simulink model "New_Control_Law_I_3Axis"  (R2016a)
settings: configuration reference "AR_Drone_ConfigSet" (kept outside this file)
values from neighbouring files (symbols this model uses):
  Accel_Calib_Gain = Simulink.Parameter    [AR_DRONE_SCRIPT.m]
  Accel_Calib_Offset = Simulink.Parameter    [AR_DRONE_SCRIPT.m]
undefined symbols (not defined in the file or in its folder): Drone_StateModeType, Mag_Calib_Gain_Vector, Mag_Calib_Offset_Vector, Navigation, Navigation_KF_Lib, sigbuilder_block
libraries: simulink x16, vrlib x7, aerolibtransform2 x5, AR_Drone_Sensors x2, AR_Drone_Actuators x2, aerolibutil x2, dspnetwork x2
(part 3 of 3)

== system New_Control_Law_I_3Axis/Sensor  Telemetry/CheckSum_Correct_Pressure/CheckSum Correction/Generate Sample Holding Pulse/Transition Logic Detection ==
  Input : Inport
  Constant : Constant  Value=0
  Constant1 : Constant
  Logical Operator : Logic  AllPortsSameDT=off  OutDataTypeStr=boolean
  Relational Operator : RelationalOperator  Operator===  OutDataTypeStr=boolean
  Relational Operator1 : RelationalOperator  Operator===  OutDataTypeStr=boolean
  Unit Delay : UnitDelay  SampleTime=-1
  Transition Detect : Outport
  wires:
  Relational Operator1/1 -> Logical Operator/1
  Unit Delay/1 -> Relational Operator/1
  Input/1 -> Relational Operator1/2, Unit Delay/1
  Relational Operator/1 -> Logical Operator/2
  Constant/1 -> Relational Operator/2
  Constant1/1 -> Relational Operator1/1
  Logical Operator/1 -> Transition Detect/1  "Transition_Detect"

== system New_Control_Law_I_3Axis/Sensor  Telemetry/CheckSum_Correct_Temp/CheckSum Correction/Generate Sample Holding Pulse/Transition Logic Detection ==
  Input : Inport
  Constant : Constant  Value=0
  Constant1 : Constant
  Logical Operator : Logic  AllPortsSameDT=off  OutDataTypeStr=boolean
  Relational Operator : RelationalOperator  Operator===  OutDataTypeStr=boolean
  Relational Operator1 : RelationalOperator  Operator===  OutDataTypeStr=boolean
  Unit Delay : UnitDelay  SampleTime=-1
  Transition Detect : Outport
  wires:
  Relational Operator1/1 -> Logical Operator/1
  Unit Delay/1 -> Relational Operator/1
  Input/1 -> Relational Operator1/2, Unit Delay/1
  Relational Operator/1 -> Logical Operator/2
  Constant/1 -> Relational Operator/2
  Constant1/1 -> Relational Operator1/1
  Logical Operator/1 -> Transition Detect/1  "Transition_Detect"

== system New_Control_Law_I_3Axis/Navigation/CheckSum Pre-Processing/Accelerometer Processing/CheckSum Correction/Generate Sample Holding Pulse/Transition Logic Detection ==
  Input : Inport
  Constant : Constant  Value=0
  Constant1 : Constant
  Logical Operator : Logic  AllPortsSameDT=off  OutDataTypeStr=boolean
  Relational Operator : RelationalOperator  Operator===  OutDataTypeStr=boolean
  Relational Operator1 : RelationalOperator  Operator===  OutDataTypeStr=boolean
  Unit Delay : UnitDelay  SampleTime=-1
  Transition Detect : Outport
  wires:
  Logical Operator/1 -> Transition Detect/1  "Transition_Detect"
  Constant1/1 -> Relational Operator1/1
  Constant/1 -> Relational Operator/2
  Relational Operator/1 -> Logical Operator/2
  Input/1 -> Unit Delay/1, Relational Operator1/2
  Unit Delay/1 -> Relational Operator/1
  Relational Operator1/1 -> Logical Operator/1

== system New_Control_Law_I_3Axis/Navigation/CheckSum Pre-Processing/Magnetometer/CheckSum Correction/Generate Sample Holding Pulse/Transition Logic Detection ==
  Input : Inport
  Constant : Constant  Value=0
  Constant1 : Constant
  Logical Operator : Logic  AllPortsSameDT=off  OutDataTypeStr=boolean
  Relational Operator : RelationalOperator  Operator===  OutDataTypeStr=boolean
  Relational Operator1 : RelationalOperator  Operator===  OutDataTypeStr=boolean
  Unit Delay : UnitDelay  SampleTime=-1
  Transition Detect : Outport
  wires:
  Logical Operator/1 -> Transition Detect/1  "Transition_Detect"
  Constant1/1 -> Relational Operator1/1
  Constant/1 -> Relational Operator/2
  Relational Operator/1 -> Logical Operator/2
  Input/1 -> Unit Delay/1, Relational Operator1/2
  Unit Delay/1 -> Relational Operator/1
  Relational Operator1/1 -> Logical Operator/1

== system New_Control_Law_I_3Axis/Navigation/CheckSum Pre-Processing/RateGyro Processing/CheckSum Correction/Generate Sample Holding Pulse/Transition Logic Detection ==
  Input : Inport
  Constant : Constant  Value=0
  Constant1 : Constant
  Logical Operator : Logic  AllPortsSameDT=off  OutDataTypeStr=boolean
  Relational Operator : RelationalOperator  Operator===  OutDataTypeStr=boolean
  Relational Operator1 : RelationalOperator  Operator===  OutDataTypeStr=boolean
  Unit Delay : UnitDelay  SampleTime=-1
  Transition Detect : Outport
  wires:
  Logical Operator/1 -> Transition Detect/1  "Transition_Detect"
  Constant1/1 -> Relational Operator1/1
  Constant/1 -> Relational Operator/2
  Relational Operator/1 -> Logical Operator/2
  Input/1 -> Unit Delay/1, Relational Operator1/2
  Unit Delay/1 -> Relational Operator/1
  Relational Operator1/1 -> Logical Operator/1

== system New_Control_Law_I_3Axis/Navigation/CheckSum Pre-Processing/TempFilter/CheckSum Correction/Generate Sample Holding Pulse/Transition Logic Detection ==
  Input : Inport
  Constant : Constant  Value=0
  Constant1 : Constant
  Logical Operator : Logic  AllPortsSameDT=off  OutDataTypeStr=boolean
  Relational Operator : RelationalOperator  Operator===  OutDataTypeStr=boolean
  Relational Operator1 : RelationalOperator  Operator===  OutDataTypeStr=boolean
  Unit Delay : UnitDelay  SampleTime=-1
  Transition Detect : Outport
  wires:
  Logical Operator/1 -> Transition Detect/1  "Transition_Detect"
  Constant1/1 -> Relational Operator1/1
  Constant/1 -> Relational Operator/2
  Relational Operator/1 -> Logical Operator/2
  Input/1 -> Unit Delay/1, Relational Operator1/2
  Unit Delay/1 -> Relational Operator/1
  Relational Operator1/1 -> Logical Operator/1

== system New_Control_Law_I_3Axis/Navigation/CheckSum Pre-Processing/Ultrasound Processing/CheckSum Correction/Generate Sample Holding Pulse/Transition Logic Detection ==
  Input : Inport
  Constant : Constant  Value=0
  Constant1 : Constant
  Logical Operator : Logic  AllPortsSameDT=off  OutDataTypeStr=boolean
  Relational Operator : RelationalOperator  Operator===  OutDataTypeStr=boolean
  Relational Operator1 : RelationalOperator  Operator===  OutDataTypeStr=boolean
  Unit Delay : UnitDelay  SampleTime=-1
  Transition Detect : Outport
  wires:
  Logical Operator/1 -> Transition Detect/1  "Transition_Detect"
  Constant1/1 -> Relational Operator1/1
  Constant/1 -> Relational Operator/2
  Relational Operator/1 -> Logical Operator/2
  Input/1 -> Unit Delay/1, Relational Operator1/2
  Unit Delay/1 -> Relational Operator/1
  Relational Operator1/1 -> Logical Operator/1

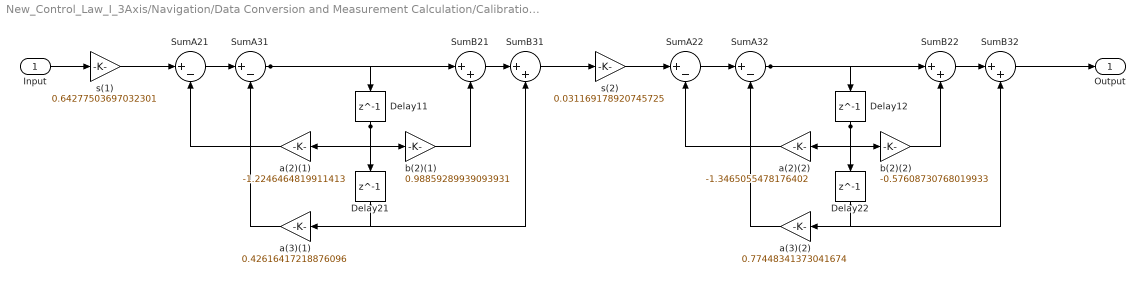
== system New_Control_Law_I_3Axis/Navigation/Data Conversion and Measurement Calculation/Calibration_Scale_and_Offset/Process Raw Mag Data/Process Raw Mag Data (Work_255725)/Low Pass Filter1 ==
  Input : Inport
  Delay{11..12,21..22} (4 alike) : Delay  DelayLength=1  InitialCondition=0
  SumA{21..22,31..32} (4 alike) : Sum  Inputs=|+-  RndMeth=Nearest  SaturateOnIntegerOverflow=on  OutDataTypeStr=Inherit: Same as first input
  SumB{21..22,31..32} (4 alike) : Sum  Inputs=|++  RndMeth=Nearest  SaturateOnIntegerOverflow=on  OutDataTypeStr=Inherit: Same as first input
  a(2)(1) : Gain  Gain=-1.2246464819911413  ParamDataTypeStr=double  RndMeth=Nearest  SaturateOnIntegerOverflow=on  OutDataTypeStr=Inherit: Same as input
  a(2)(2) : Gain  Gain=-1.3465055478176402  ParamDataTypeStr=double  RndMeth=Nearest  SaturateOnIntegerOverflow=on  OutDataTypeStr=Inherit: Same as input
  a(3)(1) : Gain  Gain=0.42616417218876096  ParamDataTypeStr=double  RndMeth=Nearest  SaturateOnIntegerOverflow=on  OutDataTypeStr=Inherit: Same as input
  a(3)(2) : Gain  Gain=0.77448341373041674  ParamDataTypeStr=double  RndMeth=Nearest  SaturateOnIntegerOverflow=on  OutDataTypeStr=Inherit: Same as input
  b(2)(1) : Gain  Gain=0.98859289939093931  ParamDataTypeStr=double  RndMeth=Nearest  SaturateOnIntegerOverflow=on  OutDataTypeStr=Inherit: Same as input
  b(2)(2) : Gain  Gain=-0.57608730768019933  ParamDataTypeStr=double  RndMeth=Nearest  SaturateOnIntegerOverflow=on  OutDataTypeStr=Inherit: Same as input
  s(1) : Gain  Gain=0.64277503697032301  ParamDataTypeStr=double  RndMeth=Nearest  SaturateOnIntegerOverflow=on  OutDataTypeStr=Inherit: Same as input
  s(2) : Gain  Gain=0.031169178920745725  ParamDataTypeStr=double  RndMeth=Nearest  SaturateOnIntegerOverflow=on  OutDataTypeStr=Inherit: Same as input
  Output : Outport
  wires:
  Delay22/1 -> SumB32/2, a(3)(2)/1
  a(3)(2)/1 -> SumA32/2
  b(2)(2)/1 -> SumB22/2
  Delay12/1 -> Delay22/1, b(2)(2)/1, a(2)(2)/1
  a(2)(2)/1 -> SumA22/2
  SumB32/1 -> Output/1
  SumB22/1 -> SumB32/1
  SumA32/1 -> Delay12/1, SumB22/1
  SumA22/1 -> SumA32/1
  s(2)/1 -> SumA22/1
  Delay21/1 -> SumB31/2, a(3)(1)/1
  a(3)(1)/1 -> SumA31/2
  b(2)(1)/1 -> SumB21/2
  Delay11/1 -> Delay21/1, b(2)(1)/1, a(2)(1)/1
  a(2)(1)/1 -> SumA21/2
  SumB31/1 -> s(2)/1
  SumB21/1 -> SumB31/1
  SumA31/1 -> Delay11/1, SumB21/1
  SumA21/1 -> SumA31/1
  s(1)/1 -> SumA21/1
  Input/1 -> s(1)/1

== stateflow chart New_Control_Law_I_3Axis/Sensor  Telemetry/CheckSum_Correct_Temp/CheckSum Correction/Generate Sample Holding Pulse/Chart ==
  state Begin_State0
    entry: output =0;
  state Begin_State
    entry: output =1;
  state End_State
    entry: output=0;
  (default) -> Begin_State0
  Begin_State0 -> Begin_State : [if_transition==1]
  Begin_State -> End_State [order 1] : after(HoldDataTicks,tick)
  End_State -> Begin_State : [if_transition==1]
  Begin_State -> Begin_State [order 2] : [if_transition==1]
  data: output output; if_transition input; HoldDataTicks input

== stateflow chart New_Control_Law_I_3Axis/Navigation/CheckSum Pre-Processing/Accelerometer Processing/CheckSum Correction/Generate Sample Holding Pulse/Chart ==
  state Begin_State0
    entry: output =0;
  state Begin_State
    entry: output =1;
  state End_State
    entry: output=0;
  (default) -> Begin_State0
  Begin_State0 -> Begin_State : [if_transition==1]
  Begin_State -> End_State [order 1] : after(HoldDataTicks,tick)
  End_State -> Begin_State : [if_transition==1]
  Begin_State -> Begin_State [order 2] : [if_transition==1]
  data: output output; if_transition input; HoldDataTicks input

== stateflow chart New_Control_Law_I_3Axis/Navigation/CheckSum Pre-Processing/RateGyro Processing/CheckSum Correction/Generate Sample Holding Pulse/Chart ==
  state Begin_State0
    entry: output =0;
  state Begin_State
    entry: output =1;
  state End_State
    entry: output=0;
  (default) -> Begin_State0
  Begin_State0 -> Begin_State : [if_transition==1]
  Begin_State -> End_State [order 1] : after(HoldDataTicks,tick)
  End_State -> Begin_State : [if_transition==1]
  Begin_State -> Begin_State [order 2] : [if_transition==1]
  data: output output; if_transition input; HoldDataTicks input

== stateflow chart New_Control_Law_I_3Axis/Sensor  Telemetry/CheckSum_Correct_Pressure/CheckSum Correction/Generate Sample Holding Pulse/Chart ==
  state Begin_State0
    entry: output =0;
  state Begin_State
    entry: output =1;
  state End_State
    entry: output=0;
  (default) -> Begin_State0
  Begin_State0 -> Begin_State : [if_transition==1]
  Begin_State -> End_State [order 1] : after(HoldDataTicks,tick)
  End_State -> Begin_State : [if_transition==1]
  Begin_State -> Begin_State [order 2] : [if_transition==1]
  data: output output; if_transition input; HoldDataTicks input

== stateflow chart New_Control_Law_I_3Axis/Navigation/CheckSum Pre-Processing/Magnetometer/CheckSum Correction/Generate Sample Holding Pulse/Chart ==
  state Begin_State0
    entry: output =0;
  state Begin_State
    entry: output =1;
  state End_State
    entry: output=0;
  (default) -> Begin_State0
  Begin_State0 -> Begin_State : [if_transition==1]
  Begin_State -> End_State [order 1] : after(HoldDataTicks,tick)
  End_State -> Begin_State : [if_transition==1]
  Begin_State -> Begin_State [order 2] : [if_transition==1]
  data: output output; if_transition input; HoldDataTicks input

== stateflow chart New_Control_Law_I_3Axis/Navigation/CheckSum Pre-Processing/Ultrasound Processing/CheckSum Correction/Generate Sample Holding Pulse/Chart ==
  state Begin_State0
    entry: output =0;
  state Begin_State
    entry: output =1;
  state End_State
    entry: output=0;
  (default) -> Begin_State0
  Begin_State0 -> Begin_State : [if_transition==1]
  Begin_State -> End_State [order 1] : after(HoldDataTicks,tick)
  End_State -> Begin_State : [if_transition==1]
  Begin_State -> Begin_State [order 2] : [if_transition==1]
  data: output output; if_transition input; HoldDataTicks input

== stateflow chart New_Control_Law_I_3Axis/Navigation/CheckSum Pre-Processing/TempFilter/CheckSum Correction/Generate Sample Holding Pulse/Chart ==
  state Begin_State0
    entry: output =0;
  state Begin_State
    entry: output =1;
  state End_State
    entry: output=0;
  (default) -> Begin_State0
  Begin_State0 -> Begin_State : [if_transition==1]
  Begin_State -> End_State [order 1] : after(HoldDataTicks,tick)
  End_State -> Begin_State : [if_transition==1]
  Begin_State -> Begin_State [order 2] : [if_transition==1]
  data: output output; if_transition input; HoldDataTicks input

== matlab function New_Control_Law_I_3Axis/Navigation/CheckSum Pre-Processing/Ultrasound Processing/Height Calculation ==
  data: u input double; y output double; prev_good_height output double; z_1 input double
function [y,prev_good_height] = fcn(u,z_1)
%#codegen



if u<10000
    
    height = ((u - 880) /26.553);
    prev_good_height = height;
else
    
%     height = u;
%     prev_good_height = height;
    height =  z_1;
    prev_good_height = z_1; 
end

y = height;

== matlab function New_Control_Law_I_3Axis/SL3D Visualization/Matrix Re-Order ==
  data: M_in input; M_out output
function M_out = MatrixFormat(M_in)
%#codegen

% SL3D coordinate system is different. This EML block is responsible for
% re-ordering the matrix in a format that SL3D can understand

M_out = M_in ; %set size

%re-order diagonal
M_out(1,1) = M_in(2,2);
M_out(2,2) = M_in(3,3);
M_out(3,3) = M_in(1,1);

%re-order bottom half
M_out(2,1) = M_in(3,2) ;
M_out(3,1) = M_in(1,2) ;
M_out(3,2) = M_in(1,3);

%re-order upper half
M_out(1,2) = M_in(2,3);
M_out(1,3) = M_in(2,1) ;
M_out(2,3) = M_in(3,1);

== stateflow chart New_Control_Law_I_3Axis/Flight Controller/Supervisory Flight Controller ==
  state Fault_Check [parallel]
    settings: executionOrder=3
    state BatteryFault_Check [parallel]
      settings: executionOrder=1
      state BatteryNominal
        en:
        BatteryFault = 0;
        state Nominal
        note: Description:
            | This state will be responsible for the following
            |
            | - Automatically land the drone by forcing it to the land state when voltage is low
            | - Prevent drone from taking off if battery voltage is too low
        state EvaluateVoltageLevel
        state ChangeState
          en:
          BatteryFault = 1;
        EvaluateVoltageLevel -> Fault_Check.BatteryFault_Check.BatteryNominal.Nominal [order 1] : [Measured_Battery_Voltage>=10.1]
        Fault_Check.BatteryFault_Check.BatteryNominal.Nominal -> EvaluateVoltageLevel : [Measured_Battery_Voltage<10.1]
        (default) -> EvaluateVoltageLevel
        EvaluateVoltageLevel -> Fault_Check.BatteryFault_Check.BatteryNominal.ChangeState [order 2] : after(5,sec)
      state BatteryLow
        state ForceLanding
          en:
        (default) -> ForceLanding
      (default) -> BatteryNominal
    state UltraSoundwarning_Check [parallel]
      settings: executionOrder=2
    state SafeOrientation_Check [parallel]
      settings: executionOrder=3
      state UnsafeOrientation
        du:
        MotorArmed =0;
        LandingPhase = 0;
      state WaitForFlight
      state GravityVectorCheck
        en:
        OrientationFault = 0;
        note: Description:
            | This state will be responsible for the following
            |
            | - Automatically land the drone by forcing it to the land state when voltage is low
            | - Prevent drone from taking off if battery voltage is too low
        state Nominal
        state EvaluateGravityVector
        state ChangeState
          en:
          OrientationFault = 1;
        EvaluateGravityVector -> Fault_Check.SafeOrientation_Check.GravityVectorCheck.Nominal [order 1] : [AccelVector_Input<-0.05]
        Fault_Check.SafeOrientation_Check.GravityVectorCheck.Nominal -> EvaluateGravityVector : [AccelVector_Input>=0.05]
        (default) -> EvaluateGravityVector
        EvaluateGravityVector -> Fault_Check.SafeOrientation_Check.GravityVectorCheck.ChangeState [order 2] : after(0.01,sec)
      (default) -> WaitForFlight
      GravityVectorCheck -> WaitForFlight : [in(Drone_State.WaitForHost)]
      WaitForFlight -> GravityVectorCheck : [in(Drone_State.Controlled_Flight)]
  state Drone_State [parallel]
    settings: executionOrder=1
    state WaitForHost
      entry:
      reset_offset_calc = 0;
      MotorArmed = 0;
      refHeight = 0;
      LandingPhase = 0;
      initDone=0;
      note: Description:
          | -This state will wait for the host command to take off
    state Initialize
      entry:
      reset_offset_calc = 0;
      MotorArmed = 0;
      refHeight = 0;
      LandingPhase = 0;
      initDone=0;
      note: Description:
          | -Upon entry, this block will set the motor to NOT ARMED (turn off integrators in controller, set safety clamp of motors to OFF)
          | -Upon entry, set the refHeight to ZERO
          | -Upon entry, reset the offset calculation such that we can re-start the averaging block
      state Attitude_Convergence_Wait
        entry,during:
        Converge_Flag = checkConvergence(GyroOffset_Parameters);
      state converge = checkConvergence(Euler_Angles) [function]
      state Calculate_Attitude_Offset
        during:
        Offset_Accel_Current =Accel_Offset_Calculation(Offset_Parameters,reset_offset_calc);
        Offset_Gyro_Current =Gyro_Offset_Calculation(GyroOffset_Parameters,reset_offset_calc);
      state Done_Initialization
        entry:
      (default) -> Attitude_Convergence_Wait
      Attitude_Convergence_Wait -> Calculate_Attitude_Offset : [Converge_Flag==1 && after(0.1,sec)]
      Calculate_Attitude_Offset -> Calculate_Attitude_Offset [order 2] : [after(4,sec)]
          | {reset_offset_calc=1;
          | Offset_Accel = Offset_Accel_Current;
          | Offset_Gyro = Offset_Gyro_Current;}
      Calculate_Attitude_Offset -> Done_Initialization [order 1] : [reset_offset_calc == 1]
          | {Accel_Offset_Calculation(Offset_Parameters,reset_offset_calc);
          | Gyro_Offset_Calculation(GyroOffset_Parameters,reset_offset_calc);}
    state Controlled_Flight
      entry:
      LandingPhase = 0; refHeight = 0; MotorArmed =1;
      note: Description:
          | -Upon entry, this block will set the motor to ARMED (enable controller integrator and motor safetey unclamped)
          | -This block will command the AR Drone to fly up to a certain height using the variable refHeight
          | -The output of refHeight should be a function of desired Altitude. The most primitive assignment is to make refHeight = DesiredAltitude, this is comparable to giving the drone a step response. Alternate methods could be giving it a smooth trajectory to follow from the ground to that particular height
          |
          | -Below is an example of what it might look like
      state Altitude_Climb_Step1
        entry: refHeight = Desired_Altitude;
      state Altitude_Climb_Step2
        entry: refHeight = Desired_Altitude;
      state Altitude_Climb_Step3
        entry: refHeight = Desired_Altitude;
      state Altitude_Climb_Step5
        entry: refHeight = Desired_Altitude;
      (default) -> Altitude_Climb_Step1
      Altitude_Climb_Step1 -> Altitude_Climb_Step2 : after(5,sec)
      Altitude_Climb_Step2 -> Altitude_Climb_Step3 : after(5,sec)
      Altitude_Climb_Step3 -> Altitude_Climb_Step5 : after(5,sec)
    state Landing_Sequence
      entry:
      note: Description:
          | -Entry into this state will occur if
          | a) Battery drops to around 10.5-10.2 Volts (needs to be experimentally validated)
          | b) Entry condition is met from the user input
          | c) Attitude is out of bounds, ie: the quad rotor has tilted it's pitch to some uncontrollable angle such as 80 degrees
          |
          | Substate goals:
          | -Descend at a controllable rate and land safely
      state Climb_down_1
        entry: refHeight =1.3;
      state Climb_down_2
        entry:
        refHeight =0.5;
      state Climb_down_3
        entry: LandingPhase=1;
      (default) -> Climb_down_1 : {N=0;}
      Climb_down_2 -> Climb_down_3 : [UltraSound_Feedback(1)<=0.5 && after(0.1,sec)]
      Climb_down_1 -> Climb_down_2 : [UltraSound_Feedback(1)<=1.3 && after(0.1,sec)]
    state Landing_Terminate
      entry:
      MotorArmed =0;
      LandingPhase = 0;
      %Catch any last state action we need to do here
      note: Description:
          | This state is optional and might not be needed. Up to you if you think having an extra state for the landing phase might be useful.. if not, delete it and consolidate it into previous state
    (default) -> WaitForHost
    Landing_Terminate -> WaitForHost : [sum(MotorCmd)==0]
    WaitForHost -> Initialize : [ (hostCmd == Drone_StateModeType.Controlled_Flight)...
        |  &&...
        |  in(Fault_Check.BatteryFault_Check.BatteryNominal.Nominal) ]
    Controlled_Flight -> Landing_Terminate [order 2] : [in(Fault_Check.SafeOrientation_Check.UnsafeOrientation)]
    Controlled_Flight -> Landing_Sequence [order 1] : [(hostCmd == ...
        | Drone_StateModeType.Landing_Sequence)...
        | ||...
        |  in(Fault_Check.BatteryFault_Check.BatteryLow) ]
    Landing_Sequence -> Landing_Terminate : [sum(MotorCmd)==0]
    Done_Initialization -> Controlled_Flight
  state Flight_Controls [parallel]
    settings: executionOrder=2
    state Attitude_Command [parallel]
      entry, during:
      Attitude_Thrust = Attitude_Control(Desired_Attitude_deg,Euler_Angles,Angular_Velocity,MotorArmed);
      settings: executionOrder=1
    state Altitude_Command [parallel]
      entry, during:
      Altitude_Thrust = Altitude_Control(UltraSound_Feedback,refHeight);
      settings: executionOrder=2
    state MotorMixing_Command [parallel]
      entry, during:
      throttle = NominalThrust+EnableAltitudeCtrl*Altitude_Thrust;
      MotorCmd = Motor_Mixing(throttle,Attitude_Thrust,LandingPhase,MotorArmed);
      settings: executionOrder=3
  state deltaThrottle = Altitude_Control(HeightFeedback,refHeight) [function]
  state controls = Attitude_Control(Desired_Attitude_Deg,EulerAngle_Feedback_Deg,RateGyro_Feedback_Deg,Motor_Armed) [function]
  state MotorCommands = Motor_Mixing(throttle,RPYCmd,LandingPhase,Motor_Armed) [function]
  data: Euler_Angles function_input double size=3; converge function_output; OffsetMeasure function_input; Reset function_input; Y function_output; OffsetMeasure function_input; Reset function_input; Y function_output; HeightFeedback function_input double size=2; refHeight function_input double size=1; deltaThrottle function_output int16; Desired_Attitude_Deg function_input double size=3; EulerAngle_Feedback_Deg function_input double size=3; RateGyro_Feedback_Deg function_input double size=3; Motor_Armed function_input double size=1; controls function_output int16 size=3; throttle function_input int16 size=1; RPYCmd function_input int16 size=3; LandingPhase function_input double size=1; MotorCommands function_output; Motor_Armed function_input double size=1; hostCmd input Enum: Drone_StateModeType; Desired_Attitude_deg input size=3; UltraSound_Feedback input size=2; initDone local; MotorCmd output size=4; throttle local int16; deltaThrottle local; height local; Euler_Angles input; Angular_Velocity input; AccelVector_Input input; hoverHeight local; NominalThrust input; EnableAltitudeCtrl input; Drone_StateMode output Enum: Drone_StateModeType; Desired_Altitude input; Measured_Battery_Voltage input; Attitude_Thrust local; Altitude_Thrust local; Converge_Flag local; reset_offset_calc local; MotorArmed local; Offset_Accel data_store_memory; LandingPhase local; N local; Offset_Parameters input size=2; GyroOffset_Parameters input size=3; Offset_Gyro data_store_memory; Offset_Gyro_Current local; Offset_Value_Current local; Offset_Accel_Current local double; BatteryFault local; OrientationFault local; BatteryFault_Mode output Enum: BatteryFault_ModeType; SafeOrientation_Mode output Enum: SafeOrientation_ModeType; refHeight output
  data hostCmd settings: description=|
      | The hostCmd can take the values 0,1 and 2.
      | 
      | 0 - default state when the drone is powered up.
      | 1 - Takeoff
      | 2 - Landing
  data UltraSound_Feedback settings: description=Ultrasound Feedback will contain data on current height (cm) and altitude rate (cm/s)
  data initDone settings: description=A flag to check whether the calibration is done.
  data NominalThrust settings: description=Nominal thrust input (approximately 60% duty cycle)
  data EnableAltitudeCtrl settings: description=A flag to enable the altitude controller
  data refHeight settings: description=Desired height at which the drone needs to hover.
  function Y = Accel_Offset_Calculation(OffsetMeasure,Reset):
    | function Y = Accel_Offset_Calculation(OffsetMeasure,Reset)
    |  
    | %Compute running average while in this state. Assumed inputs
    | %are accelerometer offset values. These values are accumulated over time
    | %and divided by the total time increment to return an average values
    | Y = [0 0]';
    | persistent A_x_sum
    | persistent A_y_sum
    | persistent Tick
    | 
    | if(isempty(A_x_sum) || Reset==1)
    |     A_x_sum = 0;
    |     A_y_sum = 0;
    |     Tick = 1;
    |         
    | else
    |     
    |     Measure_X = OffsetMeasure(1);
    |     Measure_Y = OffsetMeasure(2);
    | 
    |     A_x_sum = A_x_sum + Measure_X;
    |     A_y_sum = A_y_sum + Measure_Y;
    | 
    | 
    |     Y = [A_x_sum A_y_sum]'./Tick;
    | 
    | 
    |     Tick = Tick + 1;
    | 
    | end
    | 
    | 
    | 
    | 
    | end
  function Y = Gyro_Offset_Calculation(OffsetMeasure,Reset):
    | function Y = Gyro_Offset_Calculation(OffsetMeasure,Reset)
    |  
    | %Compute running average while in this state. Assumed inputs
    | %are gyro offset values when drone is perfectly stationary on the ground. These values are accumulated over time
    | %and divided by the total time increment to return an average values
    | Y = [0 0 0]';
    | persistent A_x_sum
    | persistent A_y_sum
    | persistent A_z_sum
    | persistent Tick
    | 
    | if(isempty(A_x_sum) || Reset==1)
    |     A_x_sum = 0;
    |     A_y_sum = 0;
    |     A_z_sum = 0;
    | 
    |     Tick = 1;
    |         
    | else
    |     
    |     Measure_X = OffsetMeasure(1);
    |     Measure_Y = OffsetMeasure(2);
    |     Measure_Z = OffsetMeasure(3);
    | 
    |     A_x_sum = A_x_sum + Measure_X;
    |     A_y_sum = A_y_sum + Measure_Y;
    |     A_z_sum = A_z_sum + Measure_Z;
    | 
    | 
    |     Y = [A_x_sum A_y_sum A_z_sum]'./Tick;
    | 
    | 
    |     Tick = Tick + 1;
    | 
    | end
    | 
    | 
    | 
    | 
    | end

== matlab function New_Control_Law_I_3Axis/Flight Controller/Supervisory Flight Controller/Attitude_Control/MATLAB Function ==
  data: error input; err_normalized output
function err_normalized = normalize_angle(error)
%#codegen

err_normalized = error;

% limit the yaw component to +/- 180 degrees
% if (error(3) > 180)    % Normalize to -180,180
%     err_normalized(3) = error(3) - 360;
% elseif(error(3) < -180)
%     err_normalized(3) = error(3) + 360;
% end

end

== matlab function New_Control_Law_I_3Axis/Navigation/SL3D Visualization/Matrix Re-Order ==
  data: M_in input; M_out output
function M_out = MatrixFormat(M_in)
%#codegen

% SL3D coordinate system is different. This EML block is responsible for
% re-ordering the matrix in a format that SL3D can understand

M_out = M_in ; %set size

%re-order diagonal
M_out(1,1) = M_in(2,2);
M_out(2,2) = M_in(3,3);
M_out(3,3) = M_in(1,1);

%re-order bottom half
M_out(2,1) = M_in(3,2) ;
M_out(3,1) = M_in(1,2) ;
M_out(3,2) = M_in(1,3);

%re-order upper half
M_out(1,2) = M_in(2,3);
M_out(1,3) = M_in(2,1) ;
M_out(2,3) = M_in(3,1);

== matlab function New_Control_Law_I_3Axis/Flight Controller/Supervisory Flight Controller/Motor_Mixing/RampDownInSpeed1 ==
  data: Cmd input; motorCmd output; stopCmd input
function motorCmd = fcn(Cmd,stopCmd)
%#codegen
persistent tempCmd;
if(isempty(tempCmd))
    tempCmd = ([0;0;0;0]);
end
if(stopCmd)
    tempCmd = tempCmd + ([1;1;1;1]*15/400);
    motorCmd = Cmd - tempCmd;
    
else
    tempCmd = ([0;0;0;0]);
    motorCmd = Cmd;
end

% if (motorCmd(1) <=0)
%         motorCmd = ([0;0;0;0]);
% end

%apply lower bounding
for i=1:4
    
if motorCmd(i)<0
    motorCmd(i) = 0;
end

end
